simulink model "sf_debouncer"  (Simulink 7.6)
settings: Solver=VariableStepDiscrete  StartTime=0.0  StopTime=6  RelTol=1e-3
settings Model: Creator=The MathWorks Inc.
settings SolverCC: InsertRTBMode=Auto
settings OptimizationCC: InitFltsAndDblsToZero=on  EfficientMapNaN2IntZero=off
settings DebuggingCC: SaveWithParameterizedLinksMsg=none  SignalResolutionControl=TryResolveAllWithWarning  MultiTaskDSMMsg=warning  MultiTaskCondExecSysMsg=none  StrictBusMsg=None
settings SFSimCC: SimParseCustomCode=off
settings RTWCC: IncludeERTFirstTime=on
settings GRTTargetCC: TargetFcnLib=ansi_tfl_tmw.mat

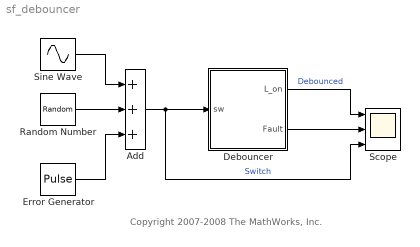
== system sf_debouncer ==
  note: Copyright 2007-2008 The MathWorks, Inc.
  Add : Sum  Inputs=+++
  Debouncer : Stateflow chart  TreatAsAtomicUnit=on
  Error Generator : DiscretePulseGenerator  PulseType=Time based  Amplitude=10  Period=0.001  PulseWidth=50  PhaseDelay=2
  Random Number : RandomNumber  Variance=30  SampleTime=0
  Scope : Scope  NumInputPorts=3
      settings: TimeRange=6.5  YMin=-1~-1~-50  YMax=1.5~1.5~50  MaxDataPoints=10000
  Sine Wave : Sin  Amplitude=20  Frequency=10  SampleTime=0
  wires:
  Debouncer/1(L_on) -> Scope/1  "Debounced"
  Sine Wave/1 -> Add/1
  Random Number/1 -> Add/2
  Add/1 -> Debouncer/1(sw), Scope/3  "Switch"
  Error Generator/1 -> Add/3
  Debouncer/2(Fault) -> Scope/2

== stateflow chart Debouncer ==
  settings: updateMethod=DISCRETE  sampleTime=0.001
  state Off
    en: L_on = 0;
    state Normal
    state Fault
      % Isolation
    (default) -> Normal
    Fault -> Normal : % Recovery
        | after(1, sec)
  state Debounce
    state On
    state Off
    Debounce.On -> Debounce.Off [order 2] : [sw < 0]
    Debounce.Off -> Debounce.On [order 2] : [sw > 0]
  state On
    en: L_on = 1;
  (default) -> Off
  Normal -> Debounce.On : [sw > 0]
  Debounce.On -> On [order 1] : after(0.1, sec)
  Debounce.Off -> Off [order 1] : after(0.1, sec)
  On -> Debounce.Off : [sw < 0]
  Debounce -> Fault : % Detection
      | after(0.3, sec)
  data: sw input double; L_on output double; Fault output unknown
